simulink model "flexcan_can_fd_slave_s32k14"  (R2017a)
settings: Solver=FixedStepDiscrete  StartTime=0.0  StopTime=10.0  FixedStep=0.1  RelTol=1e-3  EnableMultiTasking=on
InitFcn:
  | mbd_s32k14_consistency_checks(bdroot(gcs));
model workspace (MAT data in the model file):
  dt = Simulink.Parameter
  dt.Value = 0.01
  dt.DataType = 'auto'
  dt.Dimensions = [1 1]
undefined symbols (not defined in the file): A10, AD12, AD6, AD7, Aligned, B10, B8, B9, C10, C7, C8, C9, D1, D2, D8, Edge, External, G2, G3, G5, G6, H8, J8, K10, K5, K9, PTA1, PTA2, PTA3, PTB10, PTB11, PTB12, PTB8, PTB9, PTC10, PTC11, PTC12, PTC13, PTC14, PTC6, PTC7, PTD10, PTD11, PTD15, PTD16, PTD4, PTE4, PTE5, SpeedControllerIntegGain, SpeedControllerPropGain, TRGMUX_PDB_TRIG
libraries: mbd_s32k14_ec_toolbox x31, simulink x10
(part 1 of 2)
Description:
  | This model tests CAN FD for the FlexCan communication.
  | It waits for CAN FD messages with ID 0x3FF. On each received message Red LED (PTD15) is toggled.
  | 
  | HW prerequisite:
  | - S32K144EVB-Q100
  | - Make sure that J107 has pin 1 and 2 connected and external power supply is provieded through J16.
  | 
  | Validation:
  | - The CAN Baudrate is set to 500 Kb/s.
  | - Any CAN analizer (USB to CAN device) can be used to observe CAN traffic via board CAN port J13.
settings Model: Creator=agrigorev  LastModifiedBy=sreer
settings DataIOCC: ExternalInput=off  InitialState=off  LimitDataPoints=on  SaveFormat=Array  SaveOutput=off  SignalLogging=off  SaveTime=off
settings OptimizationCC: DefaultParameterBehavior=Inlined  PassReuseOutputArgsAs=Individual arguments
settings DebuggingCC: UnderspecifiedInitializationDetection=Classic  MergeDetectMultiDrivingBlocksExec=none  SolverPrmCheckMsg=warning  InheritedTsInSrcMsg=none  SingleTaskRateTransMsg=error  ParameterTunabilityLossMsg=error  UnconnectedInputMsg=error  UnconnectedOutputMsg=error  UnconnectedLineMsg=error  AllowSymbolicDim=off  UnknownTsInhSupMsg=error  StateNameClashWarn=warning  SFUnexpectedBacktrackingDiag=warning  SFNoUnconditionalDefaultTransitionDiag=warning  SFExecutionAtInitializationDiag=none
settings HardwareCC: ProdBitPerPointer=32  ProdBitPerSizeT=32  ProdBitPerPtrDiffT=32  ProdLargestAtomicInteger=Long  ProdLargestAtomicFloat=Double  ProdWordSize=32  ProdHWDeviceType=ARM Compatible->ARM Cortex
settings ModelReferenceCC: PropagateSignalLabelsOutOfModel=off
settings SFSimCC: MATLABDynamicMemAlloc=off
settings RTWCC: SystemTargetFile=mbd_s32k14.tlc  MakeCommand=mbd_s32k14_make_rtw COPY_MDLREF_INCLUDES=0  TemplateMakefile=mbd_s32k14.tmf  Description=Model Based Design Toolbox S32K14x Code Generation Target  GenerateReport=on  IncludeHyperlinkInReport=on  LaunchReport=on  GenerateTraceInfo=on  GenerateTraceReport=on  GenerateTraceReportSl=on  GenerateTraceReportSf=on  GenerateTraceReportEml=on
settings CodeAppCC: ForceParamTrailComments=on  IgnoreCustomStorageClasses=off  OperatorAnnotations=on  SimulinkDataObjDesc=on  SFDataObjDesc=on  MATLABFcnDesc=on  InsertBlockDesc=on  MATLABSourceComments=on
settings STFCustomTargetCC: MultiwordLength=256  CombineOutputUpdateFcns=on  ERTCustomFileBanners=on  SupportContinuousTime=off  SupportNonInlinedSFcns=off  RemoveResetFunc=on  MATLABClassNameForMDSCustomization=Simulink.SoftwareTarget.ERTCustomization  GRTInterface=off  SystemTargetFile=mbd_s32k14.tlc
settings ERTTargetCC: ParMdlRefBuildCompliant=off  CompOptLevelCompliant=off  ConcurrentExecutionCompliant=off  ERTFirstTimeCompliant=off  ModelStepFunctionPrototypeControlCompliant=off  CPPClassGenCompliant=off  UseToolchainInfoCompliant=off  InlinedParameterPlacement=NonHierarchical  ERTCustomFileTemplate=example_file_process.tlc
settings ConfigComp: CovMetricSettings=dw  CovHtmlReporting=on  CovSaveCumulativeToWorkspaceVar=on  CovSaveSingleToWorkspaceVar=on  CovExternalEMLEnable=off

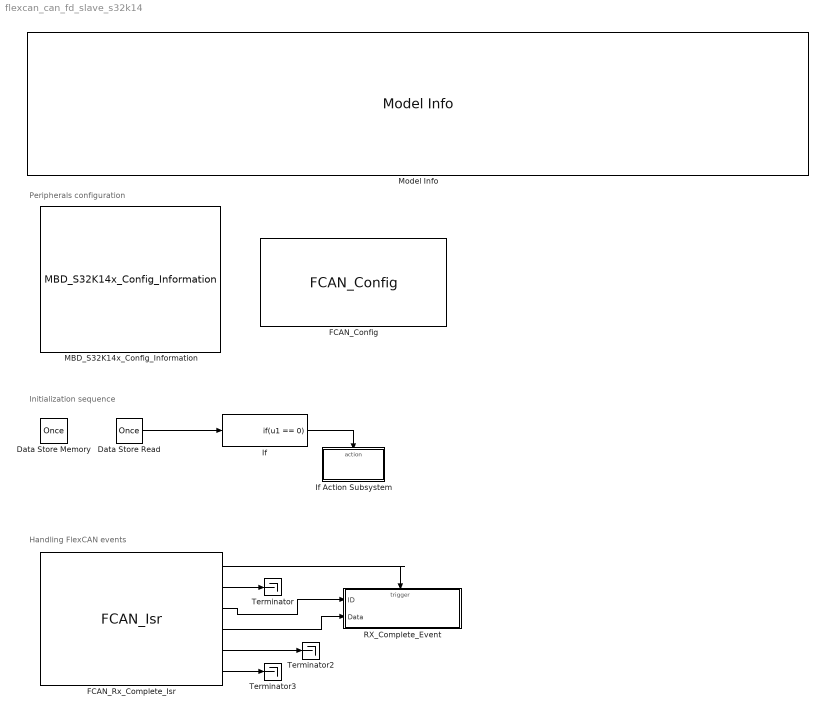
== system flexcan_can_fd_slave_s32k14 ==
  note: Initialization sequence
  note: Peripherals configuration
  note: Handling FlexCAN events
  Data Store Memory : DataStoreMemory  DataStoreName=Once  ReadBeforeWriteMsg=warning  WriteAfterWriteMsg=warning  WriteAfterReadMsg=warning  ShowAdditionalParam=off  OutDataTypeStr=uint32
  Data Store Read : DataStoreRead  DataStoreName=Once
  FCAN_Config : mbd_s32k14_ec_toolbox/S32K14x/Communication Blocks/Flex CAN Blocks/FCAN_Config  Priority=1  can_instance=0  can_mode=Normal mode  can_max_num_mb=16  can_rx=PTE4 : [9] : [6] : [D1]  can_tx=PTE5 : [8] : [5] : [D2]  show_adv_opts=on  can_clk_src=Peripheral clock  can_presdiv=9  can_rjw=0  can_pseg1=3  can_pseg2=3  can_propseg=6  can_cbt_presdiv=9  can_cbt_rjw=0  can_cbt_pseg1=3  can_cbt_pseg2=3  can_cbt_propseg=6  can_fd_enable=on  can_payload=8  can_rxfifo_enable=off  can_fifo_id_filter_extended=off  can_fifo_id_filter_remote=off  can_num_id_filters=8  can_fifo_id_format=A  can_fifo_id_filter={'0x0', '0x0', '0x0', '0x0', '0x0', '0x0', '0x0', '0x0'}  can_pn_enable=off  can_wakeup_match=off  can_wakeup_timeout=off  can_timeout_en=off  can_match_timeout=1  can_multiple_matches_en=off  can_num_matches=1  can_idfilter_extendedid=off  can_idfilter_remoteframe=off  can_idfilter_type=Match exact  can_idfilter_id1=0  can_idfilter_id2=0  can_payloadfilter_enable=off  can_payloadfilter_dlclow=0  can_payloadfilter_dlchigh=0  can_payloadfilter_type=Match exact  can_payloadfilter_payload1_b0=0  can_payloadfilter_payload1_b1=0  can_payloadfilter_payload1_b2=0  can_payloadfilter_payload1_b3=0  can_payloadfilter_payload1_b4=0  can_payloadfilter_payload1_b5=0  can_payloadfilter_payload1_b6=0  can_payloadfilter_payload1_b7=0  can_payloadfilter_payload2_b0=0  can_payloadfilter_payload2_b1=0  can_payloadfilter_payload2_b2=0  can_payloadfilter_payload2_b3=0  can_payloadfilter_payload2_b4=0  can_payloadfilter_payload2_b5=0  can_payloadfilter_payload2_b6=0  can_payloadfilter_payload2_b7=0
  FCAN_Rx_Complete_Isr : mbd_s32k14_ec_toolbox/S32K14x/Communication Blocks/Flex CAN Blocks/FCAN_Isr  can_instance=0  can_event=Rx Complete
  If : If  IfExpression=u1 == 0  ShowElse=off
  If Action Subsystem : Subsystem  TreatAsAtomicUnit=on
  MBD_S32K14x_Config_Information : mbd_s32k14_ec_toolbox/S32K14x/MBD_S32K14x_Config_Information  disp_str=|  config_params=[]
      | Target : S32K144-64KB_SRAM
      | Package : 100-pin
      | System clock : 80 MHz
      | XTAL clock : External 8 MHz
      | Compiler : GCC
      | Target Type : FLASH
      | Download Code after build : (OpenSDA: H)
      | Step Tick Interrupt Priority : 15
  Model Info : simulink/Model-Wide Utilities/Model Info  Frame=off  DisplayStringWithTags=|  HorizontalTextAlignment=Left  LeftAlignmentValue=0.02  SourceBlockDiagram=flexcan_can_fd_slave_s32k14  TagMaxNumber=20
      | Model Name: %<ModelName>
      | 
      | Description: %<Description>
  RX_Complete_Event : Subsystem  TreatAsAtomicUnit=on
      settings: RTWSystemCode=Nonreusable function
  Terminator : Terminator
  Terminator2 : Terminator
  Terminator3 : Terminator
  wires:
  If/1 -> If Action Subsystem/Action
  Data Store Read/1 -> If/1
  FCAN_Rx_Complete_Isr/5 -> Terminator2/1
  FCAN_Rx_Complete_Isr/3 -> RX_Complete_Event/1(ID)
  FCAN_Rx_Complete_Isr/2 -> Terminator/1
  FCAN_Rx_Complete_Isr/6 -> Terminator3/1
  FCAN_Rx_Complete_Isr/1 -> RX_Complete_Event/Trigger
  FCAN_Rx_Complete_Isr/4 -> RX_Complete_Event/2(Data)

== system flexcan_can_fd_slave_s32k14/If Action Subsystem ==
  Action Port : ActionPort  ActionType=then
  Constant : Constant  OutDataTypeStr=uint32
  Data Store Write : DataStoreWrite  DataStoreName=Once
  FCAN_Receive_ID_0x3FF : mbd_s32k14_ec_toolbox/S32K14x/Communication Blocks/Flex CAN Blocks/FCAN_Receive  can_instance=0  can_mode=Non-blocking  can_timeout_ms=0  can_mb_idx=14  can_extended_id=off  can_is_remote=off  can_id=3FF  can_msg_mask=FFFFFFFF  show_adv_opts=on  can_use_rxfifo=off  can_fd_enable=on
  FreeMaster_Config : mbd_s32k14_ec_toolbox/S32K14x/Utility Blocks/FreeMaster_Config  interface=UART1  baudrate=115200  rxd=PTC6 : [81] : [52] : [C7]  txd=PTC7 : [80] : [51] : [B8]  mode=Short Interrupt  isr_prio=15  show_adv_opts=off  use_scope=on  max_scope_vars=8  use_recorder=on  max_rec_vars=8  rec_buff_size=1024  rec_timebase=0 milliseconds  comm_buffer_size_auto=on  comm_buffer_size=255  comm_rqueue_size_default=on  comm_rqueue_size=32
  wires:
  Constant/1 -> Data Store Write/1

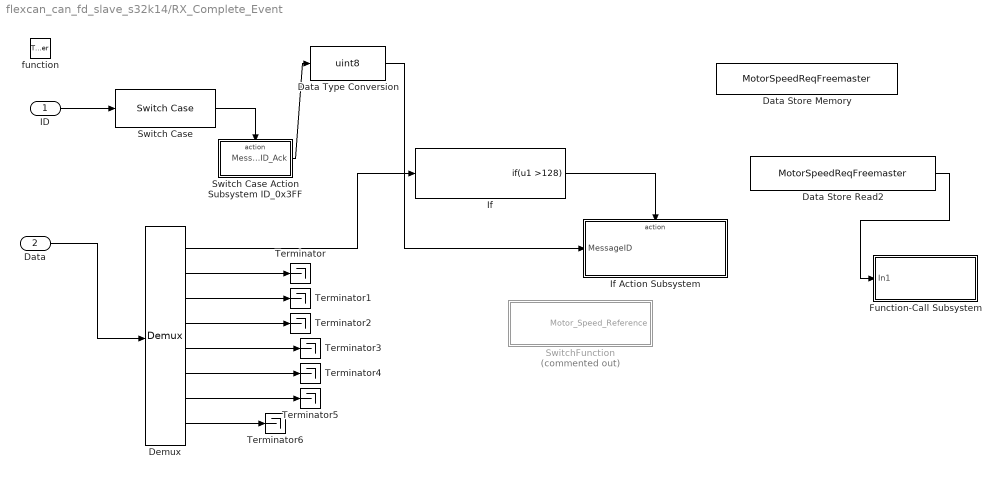
== system flexcan_can_fd_slave_s32k14/RX_Complete_Event ==
  ID : Inport
  Data : Inport  Port=2
  function : TriggerPort  TriggerType=function-call  VariantControl=Variant
  Data Store Memory : DataStoreMemory  DataStoreName=MotorSpeedReqFreemaster  ReadBeforeWriteMsg=warning  WriteAfterWriteMsg=warning  WriteAfterReadMsg=warning  ShowAdditionalParam=off  OutDataTypeStr=int16
  Data Store Read2 : DataStoreRead  DataStoreName=MotorSpeedReqFreemaster
  Data Type Conversion : DataTypeConversion  OutDataTypeStr=uint8
  Demux : Demux  Outputs=8
  Function-Call Subsystem : Subsystem  TreatAsAtomicUnit=on
  If : If  IfExpression=u1 >128  ShowElse=off
  If Action Subsystem : Subsystem  TreatAsAtomicUnit=on
  Switch Case : SwitchCase  CaseConditions={hex2dec('3FF')}  ShowDefaultCase=off
  Switch Case Action Subsystem ID_0x3FF : Subsystem  TreatAsAtomicUnit=on
  SwitchFunction : Subsystem  Commented=on  TreatAsAtomicUnit=on
  Terminator{,1..6} (7 alike) : Terminator
  wires:
  ID/1 -> Switch Case/1
  Switch Case/1 -> Switch Case Action Subsystem ID_0x3FF/Action
  Data/1 -> Demux/1
  Demux/2 -> Terminator/1
  Demux/3 -> Terminator1/1
  Demux/4 -> Terminator2/1
  Demux/5 -> Terminator3/1
  Demux/6 -> Terminator4/1
  Demux/7 -> Terminator5/1
  Demux/8 -> Terminator6/1
  If/1 -> If Action Subsystem/Action
  Data Store Read2/1 -> Function-Call Subsystem/1(In1)
  Switch Case Action Subsystem ID_0x3FF/1(MessageID_Ack) -> Data Type Conversion/1
  Demux/1 -> If/1
  Data Type Conversion/1 -> If Action Subsystem/1(MessageID)

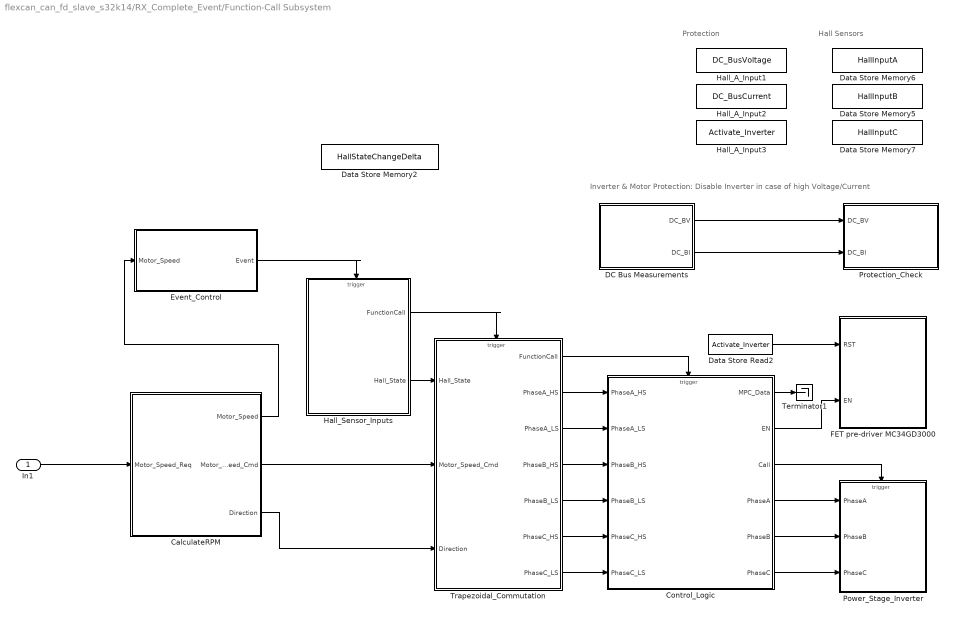
== system flexcan_can_fd_slave_s32k14/RX_Complete_Event/Function-Call Subsystem ==
  note: Inverter & Motor Protection: Disable Inverter in case of high Voltage/Current
  note: Hall Sensors
  note: Protection
  In1 : Inport
  CalculateRPM : Subsystem  TreatAsAtomicUnit=on
      settings: RTWSystemCode=Nonreusable function  RTWFcnNameOpts=Use subsystem name  RTWFileNameOpts=Use function name
  Control_Logic : Subsystem
  DC Bus Measurements : Subsystem  Priority=6
  Data Store Memory2 : DataStoreMemory  DataStoreName=HallStateChangeDelta  ReadBeforeWriteMsg=warning  WriteAfterWriteMsg=warning  WriteAfterReadMsg=warning  ShowAdditionalParam=off  OutDataTypeStr=uint16
  Data Store Memory5 : DataStoreMemory  DataStoreName=HallInputB  ReadBeforeWriteMsg=warning  WriteAfterWriteMsg=warning  WriteAfterReadMsg=warning  ShowAdditionalParam=off  OutDataTypeStr=boolean
  Data Store Memory6 : DataStoreMemory  DataStoreName=HallInputA  ReadBeforeWriteMsg=warning  WriteAfterWriteMsg=warning  WriteAfterReadMsg=warning  ShowAdditionalParam=off  OutDataTypeStr=boolean
  Data Store Memory7 : DataStoreMemory  DataStoreName=HallInputC  ReadBeforeWriteMsg=warning  WriteAfterWriteMsg=warning  WriteAfterReadMsg=warning  ShowAdditionalParam=off  OutDataTypeStr=boolean
  Data Store Read2 : DataStoreRead  DataStoreName=Activate_Inverter
  Event_Control : Subsystem  TreatAsAtomicUnit=on
      settings: RTWFcnNameOpts=Use subsystem name  RTWFileNameOpts=Use subsystem name
  FET pre-driver MC34GD3000 : Subsystem
  Hall_A_Input1 : DataStoreMemory  DataStoreName=DC_BusVoltage  ReadBeforeWriteMsg=warning  WriteAfterWriteMsg=warning  WriteAfterReadMsg=warning  ShowAdditionalParam=off  OutDataTypeStr=single
  Hall_A_Input2 : DataStoreMemory  DataStoreName=DC_BusCurrent  ReadBeforeWriteMsg=warning  WriteAfterWriteMsg=warning  WriteAfterReadMsg=warning  ShowAdditionalParam=off  OutDataTypeStr=single
  Hall_A_Input3 : DataStoreMemory  DataStoreName=Activate_Inverter  ReadBeforeWriteMsg=warning  WriteAfterWriteMsg=warning  WriteAfterReadMsg=warning  ShowAdditionalParam=off  OutDataTypeStr=boolean
  Hall_Sensor_Inputs : Subsystem
      settings: RTWFcnNameOpts=Use subsystem name  RTWFileNameOpts=Use subsystem name
  Power_Stage_Inverter : Subsystem  TreatAsAtomicUnit=on
      settings: RTWSystemCode=Nonreusable function
  Protection_Check : Subsystem
  Terminator1 : Terminator
  Trapezoidal_Commutation : Subsystem
      settings: RTWFcnNameOpts=Use subsystem name  RTWFileNameOpts=Use subsystem name
  wires:
  Control_Logic/5(PhaseB) -> Power_Stage_Inverter/2(PhaseB)
  DC Bus Measurements/1(DC_BV) -> Protection_Check/1(DC_BV)
  Control_Logic/1(MPC_Data) -> Terminator1/1
  DC Bus Measurements/2(DC_BI) -> Protection_Check/2(DC_BI)
  Control_Logic/2(EN) -> FET pre-driver MC34GD3000/2(EN)
  Trapezoidal_Commutation/6(PhaseC_HS) -> Control_Logic/5(PhaseC_HS)
  Control_Logic/4(PhaseA) -> Power_Stage_Inverter/1(PhaseA)
  Data Store Read2/1 -> FET pre-driver MC34GD3000/1(RST)
  Trapezoidal_Commutation/1(FunctionCall) -> Control_Logic/Trigger
  Trapezoidal_Commutation/4(PhaseB_HS) -> Control_Logic/3(PhaseB_HS)
  Trapezoidal_Commutation/2(PhaseA_HS) -> Control_Logic/1(PhaseA_HS)
  Trapezoidal_Commutation/7(PhaseC_LS) -> Control_Logic/6(PhaseC_LS)
  CalculateRPM/2(Motor_Speed_Cmd) -> Trapezoidal_Commutation/2(Motor_Speed_Cmd)
  CalculateRPM/3(Direction) -> Trapezoidal_Commutation/3(Direction)
  Control_Logic/6(PhaseC) -> Power_Stage_Inverter/3(PhaseC)
  CalculateRPM/1(Motor_Speed) -> Event_Control/1(Motor_Speed)
  Trapezoidal_Commutation/3(PhaseA_LS) -> Control_Logic/2(PhaseA_LS)
  Hall_Sensor_Inputs/1(FunctionCall) -> Trapezoidal_Commutation/Trigger
  Trapezoidal_Commutation/5(PhaseB_LS) -> Control_Logic/4(PhaseB_LS)
  Event_Control/1(Event) -> Hall_Sensor_Inputs/Trigger
  Hall_Sensor_Inputs/2(Hall_State) -> Trapezoidal_Commutation/1(Hall_State)
  Control_Logic/3(Call) -> Power_Stage_Inverter/Trigger
  In1/1 -> CalculateRPM/1(Motor_Speed_Req)

== system flexcan_can_fd_slave_s32k14/RX_Complete_Event/If Action Subsystem ==
  MessageID : Inport
  Action Port : ActionPort  ActionType=then
  If : If  IfExpression=u1 == 1  ShowElse=off
  If Action Subsystem : Subsystem  TreatAsAtomicUnit=on
  If Action Subsystem1 : Subsystem  Commented=on  TreatAsAtomicUnit=on
  wires:
  MessageID/1 -> If/1
  If/1 -> If Action Subsystem/Action

== system flexcan_can_fd_slave_s32k14/RX_Complete_Event/Switch Case Action Subsystem ID_0x3FF ==
  Action Port : ActionPort  ActionType=case
  Chart : Stateflow chart  TreatAsAtomicUnit=on
  FCAN_Receive_ID_0x3FF : mbd_s32k14_ec_toolbox/S32K14x/Communication Blocks/Flex CAN Blocks/FCAN_Receive  can_instance=0  can_mode=Non-blocking  can_timeout_ms=0  can_mb_idx=14  can_extended_id=off  can_is_remote=off  can_id=3FF  can_msg_mask=FFFFFFFF  show_adv_opts=on  can_use_rxfifo=off  can_fd_enable=on
  Red_LED : mbd_s32k14_ec_toolbox/S32K14x/Peripheral Interface Blocks/Digital_Output  gpio_pin=PTD15 : [22] : [15] : [G3]  port=D  pin=15  drive_strength=Low  slew_rate=Fast
  MessageID_Ack : Outport
  wires:
  Chart/1(" A") -> MessageID_Ack/1, Red_LED/1

== system flexcan_can_fd_slave_s32k14/RX_Complete_Event/SwitchFunction ==
  Chart : Stateflow chart  TreatAsAtomicUnit=on
  Data Store Memory : DataStoreMemory  DataStoreName=MotorSpeedReqFreemaster  ReadBeforeWriteMsg=warning  WriteAfterWriteMsg=warning  WriteAfterReadMsg=warning  InitialValue=1000  ShowAdditionalParam=off  OutDataTypeStr=int16
  Data Store Read1 : DataStoreRead  DataStoreName=MotorSpeedReqFreemaster
  Data Store Write : DataStoreWrite  DataStoreName=MotorSpeedReqFreemaster
  Logical Operator : Logic  Operator=NOT  AllPortsSameDT=off  OutDataTypeStr=boolean
  Logical Operator1 : Logic  Operator=NOT  AllPortsSameDT=off  OutDataTypeStr=boolean
  SW2_increment : mbd_s32k14_ec_toolbox/S32K14x/Peripheral Interface Blocks/Digital_Input  gpio_pin=PTC12 : [50] : [---] : [K9]  port=C  pin=12  pull_resistor=None  passive_filter=off
  SW3_increment : mbd_s32k14_ec_toolbox/S32K14x/Peripheral Interface Blocks/Digital_Input  gpio_pin=PTC13 : [49] : [---] : [J8]  port=C  pin=13  pull_resistor=None  passive_filter=off
  Motor_Speed_Reference : Outport
  wires:
  SW2_increment/1 -> Logical Operator1/1
  SW3_increment/1 -> Logical Operator/1
  Logical Operator1/1 -> Chart/2(Decrement)
  Logical Operator/1 -> Chart/1(Increment)
  Chart/1(out) -> Data Store Write/1
  Data Store Read1/1 -> Motor_Speed_Reference/1

== system flexcan_can_fd_slave_s32k14/RX_Complete_Event/Function-Call Subsystem/CalculateRPM ==
  Motor_Speed_Req : Inport
  Actual Motor Speed Calculation : Subsystem
  Data Store Memory1 : DataStoreMemory  DataStoreName=MechanicalRPM  ReadBeforeWriteMsg=warning  WriteAfterWriteMsg=warning  WriteAfterReadMsg=warning  ShowAdditionalParam=off  OutDataTypeStr=int16
  Data Store Read2 : DataStoreRead  DataStoreName=MechanicalRPM
  Data Store Write : DataStoreWrite  DataStoreName=MechanicalRPM
  MotorSpeedControl : Subsystem
  Motor_Speed : Outport
  Motor_Speed_Cmd : Outport  Port=2
  Direction : Outport  Port=3
  wires:
  Motor_Speed_Req/1 -> MotorSpeedControl/1(MotorSpeedReq)
  MotorSpeedControl/1(MotorSpeedCmd) -> Motor_Speed_Cmd/1
  Data Store Read2/1 -> MotorSpeedControl/2(MotorSpeedActual)
  MotorSpeedControl/2(MotorDirection) -> Actual Motor Speed Calculation/1(Direction), Direction/1
  Actual Motor Speed Calculation/1(ActualMotorSpeed) -> Data Store Write/1, Motor_Speed/1

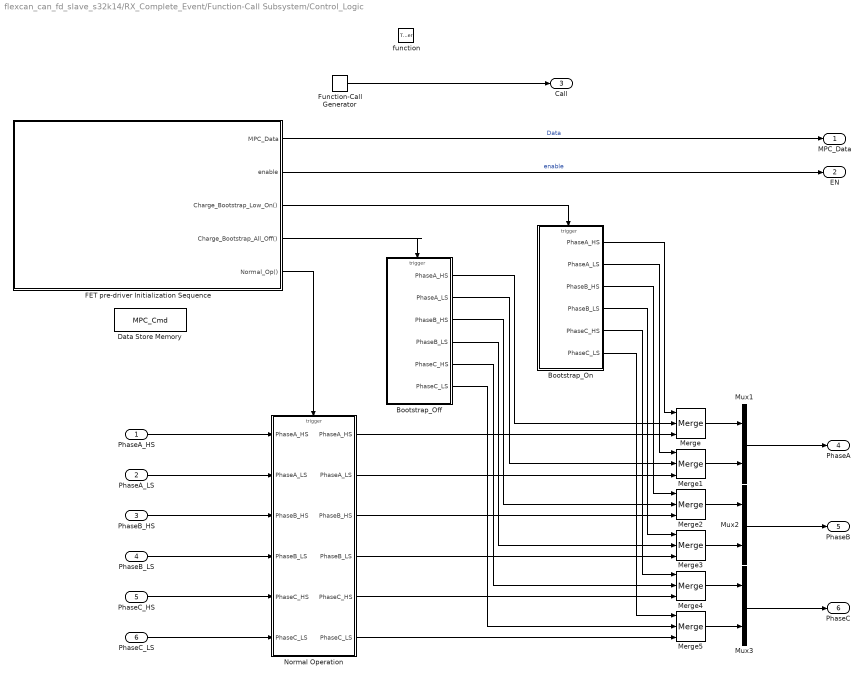
== system flexcan_can_fd_slave_s32k14/RX_Complete_Event/Function-Call Subsystem/Control_Logic ==
  PhaseA_HS : Inport
  PhaseA_LS : Inport  Port=2
  PhaseB_HS : Inport  Port=3
  PhaseB_LS : Inport  Port=4
  PhaseC_HS : Inport  Port=5
  PhaseC_LS : Inport  Port=6
  function : TriggerPort  TriggerType=function-call  VariantControl=Variant
  Bootstrap_Off : Subsystem  TreatAsAtomicUnit=on
  Bootstrap_On : Subsystem  TreatAsAtomicUnit=on
  Data Store Memory : DataStoreMemory  DataStoreName=MPC_Cmd  ReadBeforeWriteMsg=warning  WriteAfterWriteMsg=warning  WriteAfterReadMsg=warning  ShowAdditionalParam=off  OutDataTypeStr=uint8
  FET pre-driver Initialization Sequence : Stateflow chart  TreatAsAtomicUnit=on
  Function-Call Generator : simulink/Ports & Subsystems/Function-Call Generator  sample_time=-1  numberOfIterations=1
  Merge{,1..5} (6 alike) : Merge  Inputs=3
  Mux1 : Mux  Inputs=2
  Mux2 : Mux  Inputs=2
  Mux3 : Mux  Inputs=2
  Normal Operation : Subsystem  TreatAsAtomicUnit=on
  MPC_Data : Outport
  EN : Outport  Port=2
  Call : Outport  Port=3
  PhaseA : Outport  Port=4
  PhaseB : Outport  Port=5
  PhaseC : Outport  Port=6
  wires:
  Merge5/1 -> Mux3/2
  Merge2/1 -> Mux2/1
  Mux2/1 -> PhaseB/1
  Merge3/1 -> Mux2/2
  Bootstrap_Off/6(PhaseC_LS) -> Merge5/2
  Bootstrap_Off/5(PhaseC_HS) -> Merge4/2
  Bootstrap_Off/4(PhaseB_LS) -> Merge3/2
  Bootstrap_Off/3(PhaseB_HS) -> Merge2/2
  Bootstrap_Off/2(PhaseA_LS) -> Merge1/2
  Mux3/1 -> PhaseC/1
  Bootstrap_Off/1(PhaseA_HS) -> Merge/2
  Merge/1 -> Mux1/1
  Mux1/1 -> PhaseA/1
  FET pre-driver Initialization Sequence/3(Charge_Bootstrap_Low_On()) -> Bootstrap_On/Trigger
  Merge1/1 -> Mux1/2
  FET pre-driver Initialization Sequence/4(Charge_Bootstrap_All_Off()) -> Bootstrap_Off/Trigger
  Bootstrap_On/6(PhaseC_LS) -> Merge5/1
  Normal Operation/5(PhaseC_HS) -> Merge4/3
  Normal Operation/4(PhaseB_LS) -> Merge3/3
  Normal Operation/2(PhaseA_LS) -> Merge1/3
  Normal Operation/1(PhaseA_HS) -> Merge/3
  Normal Operation/6(PhaseC_LS) -> Merge5/3
  Normal Operation/3(PhaseB_HS) -> Merge2/3
  FET pre-driver Initialization Sequence/5(Normal_Op()) -> Normal Operation/Trigger
  FET pre-driver Initialization Sequence/1(MPC_Data) -> MPC_Data/1  "Data"
  FET pre-driver Initialization Sequence/2(enable) -> EN/1  "enable"
  Merge4/1 -> Mux3/1
  Bootstrap_On/5(PhaseC_HS) -> Merge4/1
  Bootstrap_On/4(PhaseB_LS) -> Merge3/1
  Bootstrap_On/3(PhaseB_HS) -> Merge2/1
  Bootstrap_On/2(PhaseA_LS) -> Merge1/1
  Bootstrap_On/1(PhaseA_HS) -> Merge/1
  PhaseA_HS/1 -> Normal Operation/1("PhaseA_HS ")
  PhaseA_LS/1 -> Normal Operation/2("PhaseA_LS ")
  PhaseB_HS/1 -> Normal Operation/3("PhaseB_HS ")
  PhaseB_LS/1 -> Normal Operation/4("PhaseB_LS ")
  PhaseC_HS/1 -> Normal Operation/5("PhaseC_HS ")
  PhaseC_LS/1 -> Normal Operation/6("PhaseC_LS ")
  Function-Call Generator/1 -> Call/1

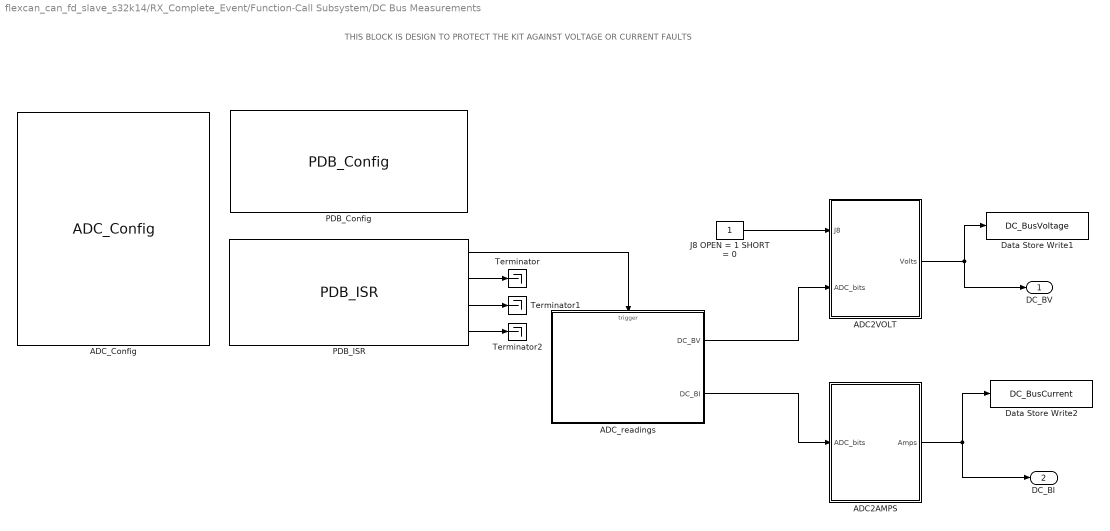
== system flexcan_can_fd_slave_s32k14/RX_Complete_Event/Function-Call Subsystem/DC Bus Measurements ==
  note: THIS BLOCK IS DESIGN TO PROTECT THE KIT AGAINST VOLTAGE OR CURRENT FAULTS
  ADC2AMPS : Subsystem
  ADC2VOLT : Subsystem
  ADC_Config : mbd_s32k14_ec_toolbox/S32K14x/Motor Control Blocks/ADC Blocks/ADC_Config  Priority=1  instance=1  mode=12-bit conversion  smplts=13  adiclk=alternate clock 1  adiv=input clock  show_adv_opts=on  pretrgsel=PDB pre-trigger  swpretrg=Disabled  adtrg=hardware  trgsel=PDB output  refsel=Vrefh and Vrefl  acfe=off  acfgt=off  acren=off  cv1=0  cv2=0  adco=off  avge=off  avgs=16 samples
  ADC_readings : Subsystem  TreatAsAtomicUnit=on
      settings: RTWSystemCode=Nonreusable function
  Data Store Write1 : DataStoreWrite  DataStoreName=DC_BusVoltage
  Data Store Write2 : DataStoreWrite  DataStoreName=DC_BusCurrent
  J8 OPEN = 1 SHORT = 0 : Constant  OutDataTypeStr=boolean
  PDB_Config : mbd_s32k14_ec_toolbox/S32K14x/Motor Control Blocks/PDB Blocks/PDB_Config  Priority=1  pdbModule=1  regScCont=Continuous  regScTrgsel=External (TRGMUX_PDB_TRIG)  trgMuxSel=FTM3 External Trigger  regModModulus=3500  regScPrescaler=1  regScMult=1  regPoenPoen0=off  regPo0DlyDly1=0  regPo0DlyDly2=1000  show_adv_opts=on  regCh0C1En0=on  regCh0C1En1=on  regCh0C1En2=off  regCh0C1En3=off  regCh0C1En4=off  regCh0C1En5=off  regCh0C1En6=off  regCh0C1En7=off  regCh0C1Bb0=off  regCh0C1Bb1=off  regCh0C1Bb2=off  regCh0C1Bb3=off  regCh0C1Bb4=off  regCh0C1Bb5=off  regCh0C1Bb6=off  regCh0C1Bb7=off  regCh0C1Tos0=Pre-trigger is in delay mode  regCh0C1Tos1=Pre-trigger is in delay mode  regCh0C1Tos2=Pre-trigger is in delay mode  regCh0C1Tos3=Pre-trigger is in delay mode  regCh0C1Tos4=Pre-trigger is in delay mode  regCh0C1Tos5=Pre-trigger is in delay mode  regCh0C1Tos6=Pre-trigger is in delay mode  regCh0C1Tos7=Pre-trigger is in delay mode  regCh0DlyDly0=1500  regCh0DlyDly1=3000  regCh0DlyDly2=100  regCh0DlyDly3=480  regCh0DlyDly4=600  regCh0DlyDly5=720  regCh0DlyDly6=840  regCh0DlyDly7=960  regCh1C1En0=off  regCh1C1En1=off  regCh1C1En2=off  regCh1C1En3=off  regCh1C1En4=off  regCh1C1En5=off  regCh1C1En6=off  regCh1C1En7=off  regCh1C1Bb0=off  regCh1C1Bb1=off  regCh1C1Bb2=off  regCh1C1Bb3=off  regCh1C1Bb4=off  regCh1C1Bb5=off  regCh1C1Bb6=off  regCh1C1Bb7=off  regCh1C1Tos0=Pre-trigger is in delay mode  regCh1C1Tos1=Pre-trigger is in delay mode  regCh1C1Tos2=Pre-trigger is in delay mode  regCh1C1Tos3=Pre-trigger is in delay mode  regCh1C1Tos4=Pre-trigger is in delay mode  regCh1C1Tos5=Pre-trigger is in delay mode  regCh1C1Tos6=Pre-trigger is in delay mode  regCh1C1Tos7=Pre-trigger is in delay mode  regCh1DlyDly0=100  regCh1DlyDly1=200  regCh1DlyDly2=300  regCh1DlyDly3=400  regCh1DlyDly4=500  regCh1DlyDly5=600  regCh1DlyDly6=700  regCh1DlyDly7=800
  PDB_ISR : mbd_s32k14_ec_toolbox/S32K14x/Motor Control Blocks/PDB Blocks/PDB_ISR  Priority=2  pdbModule=1  prioInterrupt=1  regScPdbie=on  regScPdbeie=off  regIdlyIdly=3500
  Terminator : Terminator
  Terminator1 : Terminator
  Terminator2 : Terminator
  DC_BV : Outport
  DC_BI : Outport  Port=2
  wires:
  PDB_ISR/2 -> Terminator/1
  PDB_ISR/4 -> Terminator2/1
  PDB_ISR/3 -> Terminator1/1
  PDB_ISR/1 -> ADC_readings/Trigger
  ADC2VOLT/1(Volts) -> DC_BV/1, Data Store Write1/1
  J8 OPEN = 1 SHORT = 0/1 -> ADC2VOLT/1(J8)
  ADC_readings/1(DC_BV) -> ADC2VOLT/2(ADC_bits)
  ADC2AMPS/1(Amps) -> Data Store Write2/1, DC_BI/1
  ADC_readings/2(DC_BI) -> ADC2AMPS/1(ADC_bits)

== system flexcan_can_fd_slave_s32k14/RX_Complete_Event/Function-Call Subsystem/Event_Control ==
  Motor_Speed : Inport
  ControlEventLogic : Subsystem  Priority=2
  ControlPollingLogic : Stateflow chart  TreatAsAtomicUnit=on
  HallSensorInit : Subsystem
      settings: RTWFcnNameOpts=Use subsystem name  RTWFileNameOpts=Use subsystem name
  Init : Stateflow chart  Priority=1  TreatAsAtomicUnit=on
  Mux1 : Mux  Inputs=3
  Event : Outport
  wires:
  Motor_Speed/1 -> ControlPollingLogic/1(MotorSpeedRPM)
  Mux1/1 -> Event/1
  Init/1(Init()) -> HallSensorInit/Trigger
  ControlEventLogic/1(HallStateChange) -> Mux1/3
  ControlPollingLogic/1(Trigger()) -> Mux1/2
  HallSensorInit/1(Call) -> Mux1/1

== system flexcan_can_fd_slave_s32k14/RX_Complete_Event/Function-Call Subsystem/FET pre-driver MC34GD3000 ==
  RST : Inport
  EN : Inport  Port=2
  GD3000_EN : mbd_s32k14_ec_toolbox/S32K14x/Peripheral Interface Blocks/Digital_Output  gpio_pin=PTA2 : [73] : [48] : [C10]  port=A  pin=2  drive_strength=High  slew_rate=Fast
  GD3000_RST : mbd_s32k14_ec_toolbox/S32K14x/Peripheral Interface Blocks/Digital_Output  gpio_pin="PTA3 : [72] : [47]  : [D8]"  port=A  pin=3  drive_strength=High  slew_rate=Fast
  wires:
  RST/1 -> GD3000_RST/1
  EN/1 -> GD3000_EN/1

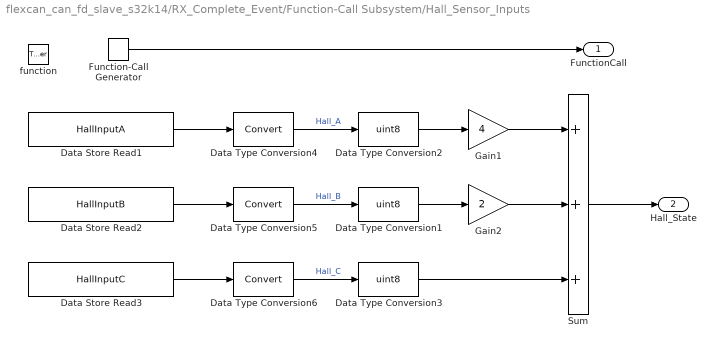
== system flexcan_can_fd_slave_s32k14/RX_Complete_Event/Function-Call Subsystem/Hall_Sensor_Inputs ==
  function : TriggerPort  TriggerType=function-call  VariantControl=Variant
  Data Store Read1 : DataStoreRead  DataStoreName=HallInputA
  Data Store Read2 : DataStoreRead  DataStoreName=HallInputB
  Data Store Read3 : DataStoreRead  DataStoreName=HallInputC
  Data Type Conversion1 : DataTypeConversion  OutDataTypeStr=uint8
  Data Type Conversion2 : DataTypeConversion  OutDataTypeStr=uint8
  Data Type Conversion3 : DataTypeConversion  OutDataTypeStr=uint8
  Data Type Conversion4 : DataTypeConversion
  Data Type Conversion5 : DataTypeConversion
  Data Type Conversion6 : DataTypeConversion
  Function-Call Generator : simulink/Ports & Subsystems/Function-Call Generator  sample_time=-1  numberOfIterations=1
  Gain1 : Gain  Gain=4  OutDataTypeStr=uint8  ParamDataTypeStr=Inherit: Same as input
  Gain2 : Gain  Gain=2  OutDataTypeStr=uint8  ParamDataTypeStr=Inherit: Same as input
  Sum : Sum  Inputs=+++  AccumDataTypeStr=uint8
  FunctionCall : Outport
  Hall_State : Outport  Port=2
  wires:
  Function-Call Generator/1 -> FunctionCall/1
  Data Store Read1/1 -> Data Type Conversion4/1
  Data Store Read2/1 -> Data Type Conversion5/1
  Data Store Read3/1 -> Data Type Conversion6/1
  Sum/1 -> Hall_State/1
  Gain1/1 -> Sum/1
  Gain2/1 -> Sum/2
  Data Type Conversion2/1 -> Gain1/1
  Data Type Conversion1/1 -> Gain2/1
  Data Type Conversion3/1 -> Sum/3
  Data Type Conversion4/1 -> Data Type Conversion2/1  "Hall_A"
  Data Type Conversion5/1 -> Data Type Conversion1/1  "Hall_B"
  Data Type Conversion6/1 -> Data Type Conversion3/1  "Hall_C"

== system flexcan_can_fd_slave_s32k14/RX_Complete_Event/Function-Call Subsystem/Power_Stage_Inverter ==
  note: NOTE
      | Phase Inputs
      | High Side is Active Low
      | Low Side is Active High
  PhaseA : Inport
  PhaseB : Inport  Port=2
  PhaseC : Inport  Port=3
  function : TriggerPort  TriggerType=function-call  VariantControl=Variant
  Demux : Demux  Outputs=2
  Demux1 : Demux  Outputs=2
  Demux2 : Demux  Outputs=2
  PWMA_HS_PWMA_LS : mbd_s32k14_ec_toolbox/S32K14x/Motor Control Blocks/FlexTimer Blocks/FTM_Independent_Output  ftmModule=3  channelPair=0-1  pwmMode=Edge-Aligned  outFrequency=20000  resolution=0.1 %  dutyCycleChN=500  dutyCycleChNP1=0  dutyCycleSim=off  startAfterInit=on  showAdvOpt=on  pinFtm0Ch0=None  pinFtm0Ch1=None  pinFtm0Ch2=None  pinFtm0Ch3=None  pinFtm0Ch4=None  pinFtm0Ch5=None  pinFtm0Ch6=None  pinFtm0Ch7=None  pinFtm1Ch0=None  pinFtm1Ch1=None  pinFtm1Ch2=None  pinFtm1Ch3=None  pinFtm1Ch4=None  pinFtm1Ch5=None  pinFtm1Ch6=None  pinFtm1Ch7=None  pinFtm2Ch0=None  pinFtm2Ch1=None  pinFtm2Ch2=None  pinFtm2Ch3=None  pinFtm2Ch4=None  pinFtm2Ch5=None  pinFtm2Ch6=None  pinFtm2Ch7=None  pinFtm3Ch0=PTB8 : [77] : [---] : [A10]  pinFtm3Ch1=PTB9 : [76] : [---] : [C8]  pinFtm3Ch2=None  pinFtm3Ch3=None  pinFtm3Ch4=None  pinFtm3Ch5=None  pinFtm3Ch6=None  pinFtm3Ch7=None  outputLevelN=Low-true pulses  outputLevelNP1=High-true pulses  initTrigger=off  chNTrigger=on  chNP1Trigger=off  mcuTargetUpdate=on
  PWMB_HS_PWMB_LS : mbd_s32k14_ec_toolbox/S32K14x/Motor Control Blocks/FlexTimer Blocks/FTM_Independent_Output  ftmModule=3  channelPair=2-3  pwmMode=Edge-Aligned  outFrequency=20000  resolution=0.1 %  dutyCycleChN=500  dutyCycleChNP1=0  dutyCycleSim=off  startAfterInit=on  showAdvOpt=off  pinFtm0Ch0=None  pinFtm0Ch1=None  pinFtm0Ch2=None  pinFtm0Ch3=None  pinFtm0Ch4=None  pinFtm0Ch5=None  pinFtm0Ch6=None  pinFtm0Ch7=None  pinFtm1Ch0=None  pinFtm1Ch1=None  pinFtm1Ch2=None  pinFtm1Ch3=None  pinFtm1Ch4=None  pinFtm1Ch5=None  pinFtm1Ch6=None  pinFtm1Ch7=None  pinFtm2Ch0=None  pinFtm2Ch1=None  pinFtm2Ch2=None  pinFtm2Ch3=None  pinFtm2Ch4=None  pinFtm2Ch5=None  pinFtm2Ch6=None  pinFtm2Ch7=None  pinFtm3Ch0=PTB8 : [77] : [---] : [A10]  pinFtm3Ch1=PTB9 : [76] : [---] : [C8]  pinFtm3Ch2=PTB10 : [75] : [---] : [B10]  pinFtm3Ch3=PTB11 : [74] : [---] : [C9]  pinFtm3Ch4=None  pinFtm3Ch5=None  pinFtm3Ch6=None  pinFtm3Ch7=None  outputLevelN=Low-true pulses  outputLevelNP1=High-true pulses  initTrigger=off  chNTrigger=off  chNP1Trigger=off  mcuTargetUpdate=on
  PWMC_HS_PWMC_LS : mbd_s32k14_ec_toolbox/S32K14x/Motor Control Blocks/FlexTimer Blocks/FTM_Independent_Output  ftmModule=3  channelPair=4-5  pwmMode=Edge-Aligned  outFrequency=20000  resolution=0.1 %  dutyCycleChN=500  dutyCycleChNP1=0  dutyCycleSim=off  startAfterInit=on  showAdvOpt=off  pinFtm0Ch0=None  pinFtm0Ch1=None  pinFtm0Ch2=None  pinFtm0Ch3=None  pinFtm0Ch4=None  pinFtm0Ch5=None  pinFtm0Ch6=None  pinFtm0Ch7=None  pinFtm1Ch0=None  pinFtm1Ch1=None  pinFtm1Ch2=None  pinFtm1Ch3=None  pinFtm1Ch4=None  pinFtm1Ch5=None  pinFtm1Ch6=None  pinFtm1Ch7=None  pinFtm2Ch0=None  pinFtm2Ch1=None  pinFtm2Ch2=None  pinFtm2Ch3=None  pinFtm2Ch4=None  pinFtm2Ch5=None  pinFtm2Ch6=None  pinFtm2Ch7=None  pinFtm3Ch0=PTB8 : [77] : [---] : [A10]  pinFtm3Ch1=PTB9 : [76] : [---] : [C8]  pinFtm3Ch2=PTB10 : [75] : [---] : [B10]  pinFtm3Ch3=PTB11 : [74] : [---] : [C9]  pinFtm3Ch4=PTC10 : [52] : [---] : [K10]  pinFtm3Ch5=PTC11 : [51] : [---] : [H8]  pinFtm3Ch6=None  pinFtm3Ch7=None  outputLevelN=Low-true pulses  outputLevelNP1=High-true pulses  initTrigger=off  chNTrigger=off  chNP1Trigger=off  mcuTargetUpdate=on
  wires:
  Demux/1 -> PWMA_HS_PWMA_LS/1
  Demux/2 -> PWMA_HS_PWMA_LS/2
  PhaseA/1 -> Demux/1
  PhaseB/1 -> Demux1/1
  Demux1/1 -> PWMB_HS_PWMB_LS/1
  Demux1/2 -> PWMB_HS_PWMB_LS/2
  PhaseC/1 -> Demux2/1
  Demux2/1 -> PWMC_HS_PWMC_LS/1
  Demux2/2 -> PWMC_HS_PWMC_LS/2

== system flexcan_can_fd_slave_s32k14/RX_Complete_Event/Function-Call Subsystem/Protection_Check ==
  DC_BV : Inport
  DC_BI : Inport  Port=2
  Abs : Abs
  FAILURE : Subsystem  TreatAsAtomicUnit=on
  If_check_Voltage_Current_limits : If  NumInputs=2  IfExpression=( (u1 > 8) & (u1 <18) ) & (u2 < 16)
  OK : Subsystem  TreatAsAtomicUnit=on
  wires:
  DC_BV/1 -> If_check_Voltage_Current_limits/1
  Abs/1 -> If_check_Voltage_Current_limits/2
  DC_BI/1 -> Abs/1
  If_check_Voltage_Current_limits/1 -> OK/Action
  If_check_Voltage_Current_limits/2 -> FAILURE/Action

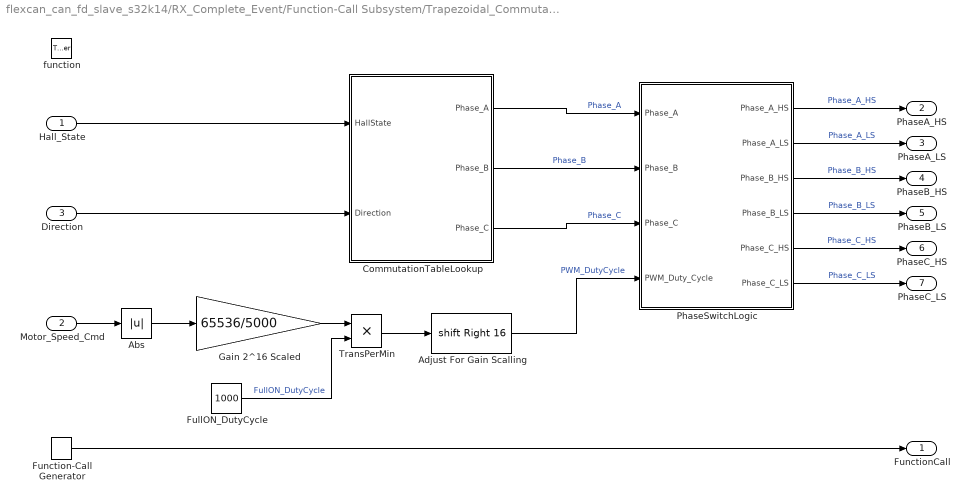
== system flexcan_can_fd_slave_s32k14/RX_Complete_Event/Function-Call Subsystem/Trapezoidal_Commutation ==
  Hall_State : Inport
  Motor_Speed_Cmd : Inport  Port=2
  Direction : Inport  Port=3
  function : TriggerPort  TriggerType=function-call  VariantControl=Variant
  Abs : Abs  OutDataTypeStr=Inherit: Inherit via internal rule
  Adjust For Gain Scalling : ArithShift  BitShiftNumber=16  BitShiftDirection=Right
  CommutationTableLookup : Stateflow chart  TreatAsAtomicUnit=on
  FullON_DutyCycle : Constant  Value=1000  OutDataTypeStr=uint16
  Function-Call Generator : simulink/Ports & Subsystems/Function-Call Generator  sample_time=-1  numberOfIterations=1
  Gain 2^16 Scaled : Gain  Gain=65536/5000  ParamDataTypeStr=uint16  OutMin=0  OutMax=100  OutDataTypeStr=uint32  RndMeth=Round  LockScale=on
  PhaseSwitchLogic : Stateflow chart  TreatAsAtomicUnit=on
  TransPerMin : Product  Inputs=**  OutDataTypeStr=Inherit: Inherit via back propagation  RndMeth=Zero
  FunctionCall : Outport
  PhaseA_HS : Outport  Port=2
  PhaseA_LS : Outport  Port=3
  PhaseB_HS : Outport  Port=4
  PhaseB_LS : Outport  Port=5
  PhaseC_HS : Outport  Port=6
  PhaseC_LS : Outport  Port=7
  wires:
  Hall_State/1 -> CommutationTableLookup/1(HallState)
  CommutationTableLookup/1(Phase_A) -> PhaseSwitchLogic/1(Phase_A)  "Phase_A"
  CommutationTableLookup/2(Phase_B) -> PhaseSwitchLogic/2(Phase_B)  "Phase_B"
  CommutationTableLookup/3(Phase_C) -> PhaseSwitchLogic/3(Phase_C)  "Phase_C"
  Abs/1 -> Gain 2^16 Scaled/1
  Function-Call Generator/1 -> FunctionCall/1
  Motor_Speed_Cmd/1 -> Abs/1
  Adjust For Gain Scalling/1 -> PhaseSwitchLogic/4(PWM_Duty_Cycle)  "PWM_DutyCycle"
  Direction/1 -> CommutationTableLookup/2(Direction)
  Gain 2^16 Scaled/1 -> TransPerMin/1
  FullON_DutyCycle/1 -> TransPerMin/2  "FullON_DutyCycle"
  TransPerMin/1 -> Adjust For Gain Scalling/1
  PhaseSwitchLogic/1(Phase_A_HS) -> PhaseA_HS/1  "Phase_A_HS"
  PhaseSwitchLogic/2(Phase_A_LS) -> PhaseA_LS/1  "Phase_A_LS"
  PhaseSwitchLogic/3(Phase_B_HS) -> PhaseB_HS/1  "Phase_B_HS"
  PhaseSwitchLogic/4(Phase_B_LS) -> PhaseB_LS/1  "Phase_B_LS"
  PhaseSwitchLogic/5(Phase_C_HS) -> PhaseC_HS/1  "Phase_C_HS"
  PhaseSwitchLogic/6(Phase_C_LS) -> PhaseC_LS/1  "Phase_C_LS"

== system flexcan_can_fd_slave_s32k14/RX_Complete_Event/If Action Subsystem/If Action Subsystem ==
  Action Port : ActionPort  ActionType=then
  Add : Sum
  Chart : Stateflow chart  TreatAsAtomicUnit=on
  Data Store Read1 : DataStoreRead  DataStoreName=MotorSpeedReqFreemaster
  Data Store Write : DataStoreWrite  DataStoreName=MotorSpeedReqFreemaster
  Logical Operator : Logic  Operator=NOT  AllPortsSameDT=off  OutDataTypeStr=boolean
  Logical Operator1 : Logic  Operator=NOT  AllPortsSameDT=off  OutDataTypeStr=boolean
  SW2_increment : mbd_s32k14_ec_toolbox/S32K14x/Peripheral Interface Blocks/Digital_Input  gpio_pin=PTC12 : [50] : [---] : [K9]  port=C  pin=12  pull_resistor=None  passive_filter=off
  SW3_increment : mbd_s32k14_ec_toolbox/S32K14x/Peripheral Interface Blocks/Digital_Input  gpio_pin=PTC13 : [49] : [---] : [J8]  port=C  pin=13  pull_resistor=None  passive_filter=off
  wires:
  Logical Operator/1 -> Chart/1(Increment)
  Logical Operator1/1 -> Chart/2(Decrement)
  SW2_increment/1 -> Logical Operator1/1
  Chart/1(out) -> Add/2
  Add/1 -> Data Store Write/1
  Data Store Read1/1 -> Add/1
  SW3_increment/1 -> Logical Operator/1

== system flexcan_can_fd_slave_s32k14/RX_Complete_Event/If Action Subsystem/If Action Subsystem1 ==
  Action Port : ActionPort
  Constant : Constant  Value=0  OutDataTypeStr=int16
  Data Store Write : DataStoreWrite  DataStoreName=MotorSpeedReqFreemaster
  wires:
  Constant/1 -> Data Store Write/1

== system flexcan_can_fd_slave_s32k14/RX_Complete_Event/Function-Call Subsystem/CalculateRPM/Actual Motor Speed Calculation ==
  Direction : Inport
  Calc_RPM1 : Subsystem
  Data Store Read2 : DataStoreRead  DataStoreName=HallStateChangeDelta
  Data Store Write1 : DataStoreWrite  DataStoreName=HallStateChangeDelta
  GatherNumberOfHallStateChanges : Stateflow chart  TreatAsAtomicUnit=on
  Saturation : Saturate  UpperLimit=5000  LowerLimit=-5000  OutDataTypeStr=int16
  ActualMotorSpeed : Outport
  wires:
  GatherNumberOfHallStateChanges/1(HallChangesSum) -> Calc_RPM1/1(HallChangeSum)
  Data Store Read2/1 -> GatherNumberOfHallStateChanges/1(HallChanges)
  GatherNumberOfHallStateChanges/2(HallChangeClear) -> Data Store Write1/1
  Direction/1 -> Calc_RPM1/2(Dir)
  Calc_RPM1/1(RPM) -> Saturation/1
  Saturation/1 -> ActualMotorSpeed/1

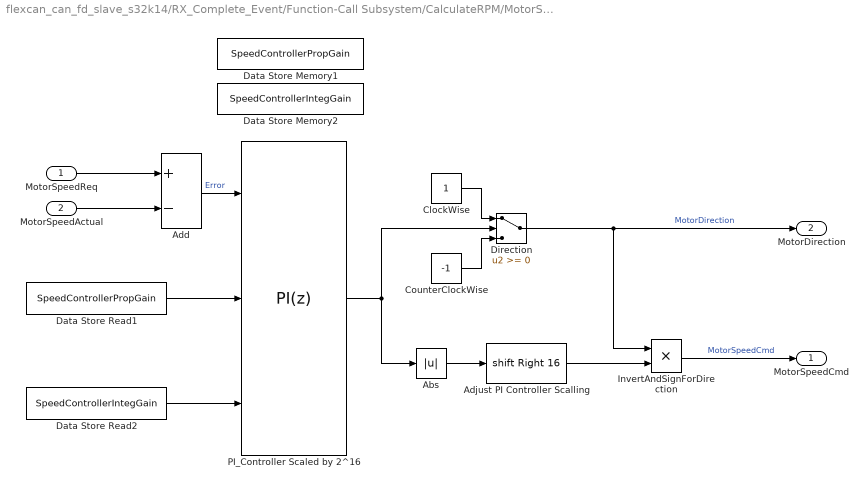
== system flexcan_can_fd_slave_s32k14/RX_Complete_Event/Function-Call Subsystem/CalculateRPM/MotorSpeedControl ==
  MotorSpeedReq : Inport
  MotorSpeedActual : Inport  Port=2
  Abs : Abs  OutDataTypeStr=uint32
  Add : Sum  Inputs=+-  AccumDataTypeStr=int32
  Adjust PI Controller Scalling : ArithShift  BitShiftNumber=16  BitShiftDirection=Right
  ClockWise : Constant  OutDataTypeStr=int8
  CounterClockWise : Constant  Value=-1  OutDataTypeStr=int8
  Data Store Memory1 : DataStoreMemory  DataStoreName=SpeedControllerPropGain  ReadBeforeWriteMsg=warning  WriteAfterWriteMsg=warning  WriteAfterReadMsg=warning  InitialValue=30000  ShowAdditionalParam=off  OutDataTypeStr=int32
  Data Store Memory2 : DataStoreMemory  DataStoreName=SpeedControllerIntegGain  ReadBeforeWriteMsg=warning  WriteAfterWriteMsg=warning  WriteAfterReadMsg=warning  InitialValue=20000  ShowAdditionalParam=off  OutDataTypeStr=int32
  Data Store Read1 : DataStoreRead  DataStoreName=SpeedControllerPropGain
  Data Store Read2 : DataStoreRead  DataStoreName=SpeedControllerIntegGain
  Direction : Switch  OutDataTypeStr=int16
  InvertAndSignForDirection : Product  Inputs=**  OutDataTypeStr=int32  RndMeth=Zero
  PI_Controller Scaled by 2^16 : simulink/Continuous/PID Controller  Controller=PI  TimeDomain=Discrete-time  SampleTime=-1  IntegratorMethod=Forward Euler  FilterMethod=Forward Euler  Form=Parallel  UseFilter=on  ControllerParametersSource=external  P=SpeedControllerPropGain  I=SpeedControllerIntegGain  D=0  N=1  InitialConditionSource=internal  InitialConditionForIntegrator=0  InitialConditionForFilter=0  ExternalReset=none  LimitOutput=on  UpperSaturationLimit=5000*65536  LowerSaturationLimit=-5000*65536  LinearizeAsGain=off  AntiWindupMode=clamping  Kb=1  TrackingMode=off  Kt=1  PParamMin=[]  PParamMax=[]  PParamDataTypeStr=int32  IParamMin=[]  IParamMax=[]  IParamDataTypeStr=int32  DParamMin=[]  DParamMax=[]  DParamDataTypeStr=single  NParamMin=[]  NParamMax=[]  NParamDataTypeStr=single  KbParamMin=[]  KbParamMax=[]  KtParamMin=[]  KtParamMax=[]  POutMin=[]  POutMax=[]  POutDataTypeStr=int32  PGainOutDataTypeStr=int32  PProdOutDataTypeStr=int32  IOutMin=[]  IOutMax=[]  IOutDataTypeStr=int32  IGainOutDataTypeStr=int32  IProdOutDataTypeStr=int32  DOutMin=[]  DOutMax=[]  DOutDataTypeStr=single  DGainOutDataTypeStr=single  DProdOutDataTypeStr=single  NOutMin=[]  NOutMax=[]  NOutDataTypeStr=single  NGainOutDataTypeStr=single  NProdOutDataTypeStr=single  KbOutMin=[]  KbOutMax=[]  KtOutMin=[]  KtOutMax=[]  IntegratorOutMin=[]  IntegratorOutMax=[]  IntegratorOutDataTypeStr=int32  FilterOutMin=[]  FilterOutMax=[]  FilterOutDataTypeStr=int32  SumOutMin=[]  SumOutMax=[]  SumOutDataTypeStr=int32  SumI1OutMin=[]  SumI1OutMax=[]  SumI2OutMin=[]  SumI2OutMax=[]  SumI3OutMin=[]  SumI3OutMax=[]  SumDOutMin=[]  SumDOutMax=[]  SumDOutDataTypeStr=single  SumAccumDataTypeStr=int32  SumDAccumDataTypeStr=single  SaturationOutMin=[]  SaturationOutMax=[]  SaturationOutDataTypeStr=int32  IntegratorContinuousStateAttributes=''  IntegratorStateMustResolveToSignalObject=off  IntegratorRTWStateStorageClass=Auto  FilterContinuousStateAttributes=''  FilterStateMustResolveToSignalObject=off  FilterRTWStateStorageClass=Auto  DifferentiatorICPrevScaledInput=0  DifferentiatorOutMin=[]  DifferentiatorOutMax=[]  InitialConditionSetting=State (most efficient)
  MotorSpeedCmd : Outport
  MotorDirection : Outport  Port=2
  wires:
  MotorSpeedActual/1 -> Add/2
  Add/1 -> PI_Controller Scaled by 2^16/1  "Error"
  Adjust PI Controller Scalling/1 -> InvertAndSignForDirection/2
  Abs/1 -> Adjust PI Controller Scalling/1
  ClockWise/1 -> Direction/1
  CounterClockWise/1 -> Direction/3
  Direction/1 -> MotorDirection/1, InvertAndSignForDirection/1  "MotorDirection"
  PI_Controller Scaled by 2^16/1 -> Direction/2, Abs/1
  InvertAndSignForDirection/1 -> MotorSpeedCmd/1  "MotorSpeedCmd"
  MotorSpeedReq/1 -> Add/1
  Data Store Read2/1 -> PI_Controller Scaled by 2^16/3
  Data Store Read1/1 -> PI_Controller Scaled by 2^16/2

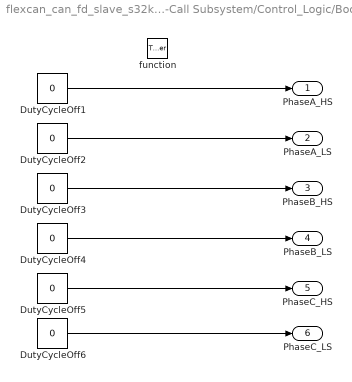
== system flexcan_can_fd_slave_s32k14/RX_Complete_Event/Function-Call Subsystem/Control_Logic/Bootstrap_Off ==
  function : TriggerPort  TriggerType=function-call  VariantControl=Variant
  DutyCycleOff{1..6} (6 alike) : Constant  Value=0  OutDataTypeStr=uint32  SampleTime=-1
  PhaseA_HS : Outport  InitialOutput=0
  PhaseA_LS : Outport  Port=2  InitialOutput=0
  PhaseB_HS : Outport  Port=3  InitialOutput=0
  PhaseB_LS : Outport  Port=4  InitialOutput=0
  PhaseC_HS : Outport  Port=5  InitialOutput=0
  PhaseC_LS : Outport  Port=6  InitialOutput=0
  wires:
  DutyCycleOff1/1 -> PhaseA_HS/1
  DutyCycleOff2/1 -> PhaseA_LS/1
  DutyCycleOff3/1 -> PhaseB_HS/1
  DutyCycleOff4/1 -> PhaseB_LS/1
  DutyCycleOff5/1 -> PhaseC_HS/1
  DutyCycleOff6/1 -> PhaseC_LS/1

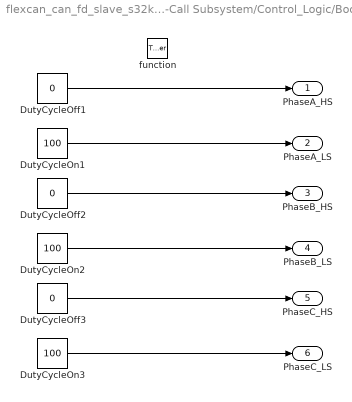
== system flexcan_can_fd_slave_s32k14/RX_Complete_Event/Function-Call Subsystem/Control_Logic/Bootstrap_On ==
  function : TriggerPort  TriggerType=function-call  VariantControl=Variant
  DutyCycleOff1 : Constant  Value=0  OutDataTypeStr=uint32  SampleTime=-1
  DutyCycleOff2 : Constant  Value=0  OutDataTypeStr=uint32  SampleTime=-1
  DutyCycleOff3 : Constant  Value=0  OutDataTypeStr=uint32  SampleTime=-1
  DutyCycleOn1 : Constant  Value=100  OutDataTypeStr=uint32  SampleTime=-1
  DutyCycleOn2 : Constant  Value=100  OutDataTypeStr=uint32  SampleTime=-1
  DutyCycleOn3 : Constant  Value=100  OutDataTypeStr=uint32  SampleTime=-1
  PhaseA_HS : Outport  InitialOutput=0
  PhaseA_LS : Outport  Port=2  InitialOutput=0
  PhaseB_HS : Outport  Port=3  InitialOutput=0
  PhaseB_LS : Outport  Port=4  InitialOutput=0
  PhaseC_HS : Outport  Port=5  InitialOutput=0
  PhaseC_LS : Outport  Port=6  InitialOutput=0
  wires:
  DutyCycleOff1/1 -> PhaseA_HS/1
  DutyCycleOn1/1 -> PhaseA_LS/1
  DutyCycleOn2/1 -> PhaseB_LS/1
  DutyCycleOn3/1 -> PhaseC_LS/1
  DutyCycleOff2/1 -> PhaseB_HS/1
  DutyCycleOff3/1 -> PhaseC_HS/1

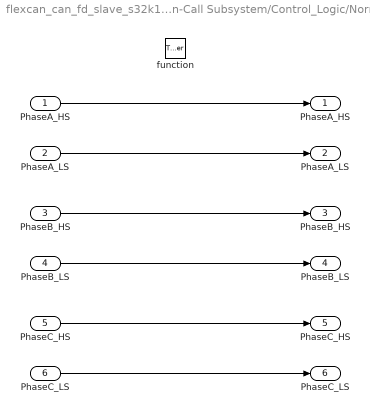
== system flexcan_can_fd_slave_s32k14/RX_Complete_Event/Function-Call Subsystem/Control_Logic/Normal Operation ==
  "PhaseA_HS " : Inport
  "PhaseA_LS " : Inport  Port=2
  "PhaseB_HS " : Inport  Port=3
  "PhaseB_LS " : Inport  Port=4
  "PhaseC_HS " : Inport  Port=5
  "PhaseC_LS " : Inport  Port=6
  function : TriggerPort  TriggerType=function-call  VariantControl=Variant
  PhaseA_HS : Outport  InitialOutput=0
  PhaseA_LS : Outport  Port=2  InitialOutput=0
  PhaseB_HS : Outport  Port=3  InitialOutput=0
  PhaseB_LS : Outport  Port=4  InitialOutput=0
  PhaseC_HS : Outport  Port=5  InitialOutput=0
  PhaseC_LS : Outport  Port=6  InitialOutput=0
  wires:
  "PhaseA_HS "/1 -> PhaseA_HS/1
  "PhaseA_LS "/1 -> PhaseA_LS/1
  "PhaseB_HS "/1 -> PhaseB_HS/1
  "PhaseB_LS "/1 -> PhaseB_LS/1
  "PhaseC_HS "/1 -> PhaseC_HS/1
  "PhaseC_LS "/1 -> PhaseC_LS/1

== system flexcan_can_fd_slave_s32k14/RX_Complete_Event/Function-Call Subsystem/DC Bus Measurements/ADC2AMPS ==
  ADC_bits : Inport
  Sum : Sum  Inputs=+-  OutDataTypeStr=single
  bits2amps : Gain  Gain=25/4095  OutDataTypeStr=single
  offset : Constant  Value=2048  OutDataTypeStr=uint32
  Amps : Outport
  wires:
  Sum/1 -> bits2amps/1
  bits2amps/1 -> Amps/1
  offset/1 -> Sum/2
  ADC_bits/1 -> Sum/1

== system flexcan_can_fd_slave_s32k14/RX_Complete_Event/Function-Call Subsystem/DC Bus Measurements/ADC2VOLT ==
  J8 : Inport
  ADC_bits : Inport  Port=2
  DC_sensing_29.75 : Constant  Value=29.75  OutDataTypeStr=single
  DC_sensing_45V : Constant  Value=45  OutDataTypeStr=single
  Product : Product  OutDataTypeStr=single
  Switch1 : Switch  Criteria=u2 > Threshold
  bits2volts : Gain  Gain=1/4095  OutDataTypeStr=single
  Volts : Outport
  wires:
  bits2volts/1 -> Volts/1
  DC_sensing_45V/1 -> Switch1/1
  DC_sensing_29.75/1 -> Switch1/3
  Product/1 -> bits2volts/1
  J8/1 -> Switch1/2
  Switch1/1 -> Product/1
  ADC_bits/1 -> Product/2

== system flexcan_can_fd_slave_s32k14/RX_Complete_Event/Function-Call Subsystem/DC Bus Measurements/ADC_readings ==
  function : TriggerPort  TriggerType=function-call  VariantControl=Variant
  Read_DC_Current : mbd_s32k14_ec_toolbox/S32K14x/Motor Control Blocks/ADC Blocks/ADC_Start  instance=1  adc_r=B  adc0_chan=PTC14 : [46] : [30] : [G6] : AD12  adc1_chan=PTD4 : [69] : [44] : [E10] : AD6  aien=off  mcuTargetUpdate=on
  Read_DC_Voltage : mbd_s32k14_ec_toolbox/S32K14x/Motor Control Blocks/ADC Blocks/ADC_Start  instance=1  adc_r=A  adc0_chan=PTC14 : [46] : [30] : [G6] : AD12  adc1_chan=PTB12 : [68] : [43] : [E9] : AD7  aien=off  mcuTargetUpdate=on
  DC_BV : Outport
  DC_BI : Outport  Port=2
  wires:
  Read_DC_Voltage/1 -> DC_BV/1
  Read_DC_Current/1 -> DC_BI/1

== system flexcan_can_fd_slave_s32k14/RX_Complete_Event/Function-Call Subsystem/Event_Control/ControlEventLogic ==
  Digital_Input_ISR_HALL_A : mbd_s32k14_ec_toolbox/S32K14x/Peripheral Interface Blocks/Digital_Input_ISR  gpio_pin=PTD11 : [35] : [---] : [G5]  port=D  pin=11  irqc=on either-edge  prio=10
  Digital_Input_ISR_HALL_B : mbd_s32k14_ec_toolbox/S32K14x/Peripheral Interface Blocks/Digital_Input_ISR  gpio_pin=PTD10 : [36] : [---] : [K5]  port=D  pin=10  irqc=on either-edge  prio=10
  Digital_Input_ISR_HALL_C : mbd_s32k14_ec_toolbox/S32K14x/Peripheral Interface Blocks/Digital_Input_ISR  gpio_pin=PTA1 : [78] : [49] : [B9]  port=A  pin=1  irqc=on either-edge  prio=10
  HallChangeCount : Subsystem
  Mux2 : Mux  Inputs=3
  ToggleLED_HallA : Subsystem
  ToggleLED_HallB : Subsystem
  ToggleLED_HallC : Subsystem
  HallStateChange : Outport
  wires:
  Mux2/1 -> HallChangeCount/Trigger
  HallChangeCount/1(Call) -> HallStateChange/1
  Digital_Input_ISR_HALL_C/1 -> ToggleLED_HallC/Trigger
  Digital_Input_ISR_HALL_B/1 -> ToggleLED_HallB/Trigger
  ToggleLED_HallB/1(Call) -> Mux2/2
  Digital_Input_ISR_HALL_A/1 -> ToggleLED_HallA/Trigger
  ToggleLED_HallA/1(Call) -> Mux2/1
  ToggleLED_HallC/1(Call) -> Mux2/3

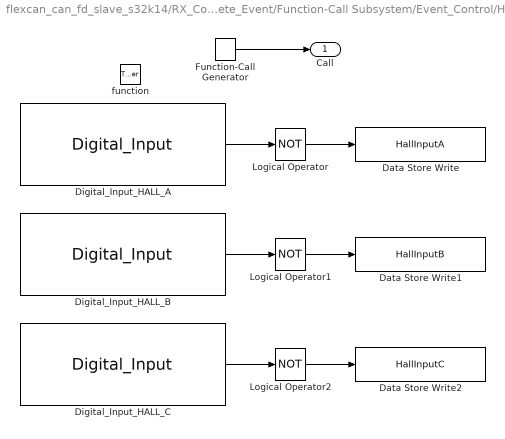
== system flexcan_can_fd_slave_s32k14/RX_Complete_Event/Function-Call Subsystem/Event_Control/HallSensorInit ==
  function : TriggerPort  TriggerType=function-call  VariantControl=Variant
  Data Store Write : DataStoreWrite  DataStoreName=HallInputA
  Data Store Write1 : DataStoreWrite  DataStoreName=HallInputB
  Data Store Write2 : DataStoreWrite  DataStoreName=HallInputC
  Digital_Input_HALL_A : mbd_s32k14_ec_toolbox/S32K14x/Peripheral Interface Blocks/Digital_Input  gpio_pin=PTD11 : [35] : [---] : [G5]  port=D  pin=11  pull_resistor=None  passive_filter=off
  Digital_Input_HALL_B : mbd_s32k14_ec_toolbox/S32K14x/Peripheral Interface Blocks/Digital_Input  gpio_pin=PTD10 : [36] : [---] : [K5]  port=D  pin=10  pull_resistor=None  passive_filter=off
  Digital_Input_HALL_C : mbd_s32k14_ec_toolbox/S32K14x/Peripheral Interface Blocks/Digital_Input  gpio_pin=PTA1 : [78] : [49] : [B9]  port=A  pin=1  pull_resistor=None  passive_filter=off
  Function-Call Generator : simulink/Ports & Subsystems/Function-Call Generator  sample_time=-1  numberOfIterations=1
  Logical Operator : Logic  Operator=NOT  AllPortsSameDT=off  OutDataTypeStr=boolean
  Logical Operator1 : Logic  Operator=NOT  AllPortsSameDT=off  OutDataTypeStr=boolean
  Logical Operator2 : Logic  Operator=NOT  AllPortsSameDT=off  OutDataTypeStr=boolean
  Call : Outport
  wires:
  Digital_Input_HALL_A/1 -> Logical Operator/1
  Digital_Input_HALL_B/1 -> Logical Operator1/1
  Digital_Input_HALL_C/1 -> Logical Operator2/1
  Function-Call Generator/1 -> Call/1
  Logical Operator/1 -> Data Store Write/1
  Logical Operator1/1 -> Data Store Write1/1
  Logical Operator2/1 -> Data Store Write2/1

== system flexcan_can_fd_slave_s32k14/RX_Complete_Event/Function-Call Subsystem/Protection_Check/FAILURE ==
  Action Port : ActionPort  ActionType=else
  Data Store Write1 : DataStoreWrite  DataStoreName=Activate_Inverter
  GREEN : mbd_s32k14_ec_toolbox/S32K14x/Peripheral Interface Blocks/Digital_Output  gpio_pin=PTD16 : [21] : [14] : [G2]  port=D  pin=16  drive_strength=Low  slew_rate=Fast
  OFF : Constant  OutDataTypeStr=boolean
  ON : Constant  Value=0  OutDataTypeStr=boolean
  ON_RST : Constant  Value=0  OutDataTypeStr=boolean
  RED : mbd_s32k14_ec_toolbox/S32K14x/Peripheral Interface Blocks/Digital_Output  gpio_pin=PTD15 : [22] : [15] : [G3]  port=D  pin=15  drive_strength=Low  slew_rate=Fast
  wires:
  ON/1 -> RED/1
  ON_RST/1 -> Data Store Write1/1
  OFF/1 -> GREEN/1

== system flexcan_can_fd_slave_s32k14/RX_Complete_Event/Function-Call Subsystem/Protection_Check/OK ==
  Action Port : ActionPort  ActionType=then
  Data Store Write1 : DataStoreWrite  DataStoreName=Activate_Inverter
  GREEN : mbd_s32k14_ec_toolbox/S32K14x/Peripheral Interface Blocks/Digital_Output  gpio_pin=PTD16 : [21] : [14] : [G2]  port=D  pin=16  drive_strength=Low  slew_rate=Fast
  OFF : Constant  OutDataTypeStr=boolean
  ON : Constant  Value=0  OutDataTypeStr=boolean
  ON_RST : Constant  OutDataTypeStr=boolean
  RED : mbd_s32k14_ec_toolbox/S32K14x/Peripheral Interface Blocks/Digital_Output  gpio_pin=PTD15 : [22] : [15] : [G3]  port=D  pin=15  drive_strength=Low  slew_rate=Fast
  wires:
  ON/1 -> GREEN/1
  ON_RST/1 -> Data Store Write1/1
  OFF/1 -> RED/1

== system flexcan_can_fd_slave_s32k14/RX_Complete_Event/Function-Call Subsystem/CalculateRPM/Actual Motor Speed Calculation/Calc_RPM1 ==
  note: Multiply by time constant to get Second
      | Mulitply by 60 to get Minute
      | Divide By State Changes to get Electrical RPM
      | Divide By Pole-Pair to get Mechanical RPM
  HallChangeSum : Inport
  Dir : Inport  Port=2
  GetDirection : Product  Inputs=**  OutDataTypeStr=int16  RndMeth=Zero
  State Changes to RPM Constant : Constant  Value=((1/(dt*250))*60)/(6*4)  OutDataTypeStr=uint16
  TransPerMin : Product  Inputs=**  OutDataTypeStr=uint16  RndMeth=Zero
  RPM : Outport
  wires:
  Dir/1 -> GetDirection/2
  GetDirection/1 -> RPM/1  "MotorSpeedRPM"
  State Changes to RPM Constant/1 -> TransPerMin/2
  HallChangeSum/1 -> TransPerMin/1
  TransPerMin/1 -> GetDirection/1

== system flexcan_can_fd_slave_s32k14/RX_Complete_Event/Function-Call Subsystem/Event_Control/ControlEventLogic/HallChangeCount ==
  function : TriggerPort  TriggerType=function-call  VariantControl=Variant
  Constant5 : Constant  OutDataTypeStr=uint16
  Data Store Read : DataStoreRead  DataStoreName=HallStateChangeDelta
  Data Store Write : DataStoreWrite  DataStoreName=HallStateChangeDelta
  Function-Call Generator : simulink/Ports & Subsystems/Function-Call Generator  sample_time=-1  numberOfIterations=1
  Increment : Sum
  Call : Outport
  wires:
  Increment/1 -> Data Store Write/1
  Constant5/1 -> Increment/1
  Data Store Read/1 -> Increment/2
  Function-Call Generator/1 -> Call/1
